simulink model "JointSpaceControl_own_MCP"  (R2013a)
settings: Solver=ode45  StartTime=0.0  StopTime=sim_end  MaxStep=0.008  RelTol=1e-3
PreLoadFcn:
  | Initialization
InitFcn:
  | Initialization
values from neighbouring files (symbols this model uses):
  a_max = [27 27 27 27 27 27]    [Initialization.m]
  dq_0 = qd_actual.signals.values(1,:)    [Initialization.m]
  K_0 = [            omega_1, zeros(1,5);         0,          omega_2, zeros(1,4);         zeros(1,2), omega_3, zeros(1,3);         zeros(1,3), omega_4, zeros(1,2);         zeros(1,4), omega_5, 0;         zeros(1,5), omega_6]    [Initialization.m]
  K_1 = [            omega_7, zeros(1,5);         0,          omega_8, zeros(1,4);         zeros(1,2), omega_9, zeros(1,3);         zeros(1,3), omega_10, zeros(1,2);         zeros(1,4), omega_11, 0;         zeros(1,5), omega_12]    [Initialization.m]
  q_0 = q_actual.signals.values(1,:)    [Initialization.m]
  q_max = 2*pi*ones(1,6)    [Initialization.m]
  q_min = -2*pi*ones(1,6)    [Initialization.m]
  torque_max = [150 150 150 28 28 28]    [Initialization.m]
  v_max = 3.4*ones(1,6)    [Initialization.m]
(part 2 of 4)

== matlab function JointSpaceControl_own_MCP/Forward & Velocity Kinematics Joint -> Tool Geometric Jacobian/J (made by Kathi) ==
  data: J output; q input; J1 output; J2 output
function [J, J1, J2]    = Jacobian(q)
% JACOBIAN - Jacobian from Base to Tool.
%  Calculates the Base-Tool Transformation matrix based on the current
%  joint positions and returns the rotation matrix and the displacement
%  vector.

theta_1 = q(1);
theta_2 = q(2);
theta_3 = q(3);
theta_4 = q(4);
theta_5 = q(5);
theta_6 = q(6);

J = [(109*cos(theta_1))/1000 + (41*cos(theta_1)*cos(theta_5))/500 + ...
        (17*cos(theta_2)*sin(theta_1))/40 - ...
        (93*cos(theta_4)*(cos(theta_2)*sin(theta_1)*sin(theta_3) + ...
        cos(theta_3)*sin(theta_1)*sin(theta_2)))/1000 + ...
        (93*sin(theta_4)*(sin(theta_1)*sin(theta_2)*sin(theta_3) - ...
        cos(theta_2)*cos(theta_3)*sin(theta_1)))/1000 - ...
        (41*sin(theta_5)*(cos(theta_4)*(sin(theta_1)*sin(theta_2)*sin(theta_3) - ...
        cos(theta_2)*cos(theta_3)*sin(theta_1)) + ...
        sin(theta_4)*(cos(theta_2)*sin(theta_1)*sin(theta_3) + ...
        cos(theta_3)*sin(theta_1)*sin(theta_2))))/500 - ...
        (39243*sin(theta_1)*sin(theta_2)*sin(theta_3))/100000 + ...
        (39243*cos(theta_2)*cos(theta_3)*sin(theta_1))/100000, ...
        ...
        (17*cos(theta_1)*sin(theta_2))/40 - ...
        (93*cos(theta_4)*(cos(theta_1)*sin(theta_2)*sin(theta_3) - ...
        cos(theta_1)*cos(theta_2)*cos(theta_3)))/1000 - ...
        (93*sin(theta_4)*(cos(theta_1)*cos(theta_2)*sin(theta_3) + ...
        cos(theta_1)*cos(theta_3)*sin(theta_2)))/1000 + ...
        (41*sin(theta_5)*(cos(theta_4)*(cos(theta_1)*cos(theta_2)*sin(theta_3) + ...
        cos(theta_1)*cos(theta_3)*sin(theta_2)) - ...
        sin(theta_4)*(cos(theta_1)*sin(theta_2)*sin(theta_3) - ...
        cos(theta_1)*cos(theta_2)*cos(theta_3))))/500 + ...
        (39243*cos(theta_1)*cos(theta_2)*sin(theta_3))/100000 + ...
        (39243*cos(theta_1)*cos(theta_3)*sin(theta_2))/100000, ...
        ...
        (41*sin(theta_5)*(cos(theta_4)*(cos(theta_1)*cos(theta_2)*sin(theta_3) + ...
        cos(theta_1)*cos(theta_3)*sin(theta_2)) - ...
        sin(theta_4)*(cos(theta_1)*sin(theta_2)*sin(theta_3) - ...
        cos(theta_1)*cos(theta_2)*cos(theta_3))))/500 - ...
        (93*sin(theta_4)*(cos(theta_1)*cos(theta_2)*sin(theta_3) + ...
        cos(theta_1)*cos(theta_3)*sin(theta_2)))/1000 - ...
        (93*cos(theta_4)*(cos(theta_1)*sin(theta_2)*sin(theta_3) - ...
        cos(theta_1)*cos(theta_2)*cos(theta_3)))/1000 + ...
        (39243*cos(theta_1)*cos(theta_2)*sin(theta_3))/100000 + ...
        (39243*cos(theta_1)*cos(theta_3)*sin(theta_2))/100000, ...
        ...
        (41*sin(theta_5)*(cos(theta_4)*(cos(theta_1)*cos(theta_2)*sin(theta_3) + ...
        cos(theta_1)*cos(theta_3)*sin(theta_2)) - ...
        sin(theta_4)*(cos(theta_1)*sin(theta_2)*sin(theta_3) - ...
        cos(theta_1)*cos(theta_2)*cos(theta_3))))/500 - ...
        (93*sin(theta_4)*(cos(theta_1)*cos(theta_2)*sin(theta_3) + ...
        cos(theta_1)*cos(theta_3)*sin(theta_2)))/1000 - ...
        (93*cos(theta_4)*(cos(theta_1)*sin(theta_2)*sin(theta_3) - ...
        cos(theta_1)*cos(theta_2)*cos(theta_3)))/1000, ...
        ...
        (41*cos(theta_5)*(cos(theta_4)*(cos(theta_1)*sin(theta_2)*sin(theta_3) - ...
        cos(theta_1)*cos(theta_2)*cos(theta_3)) + ...
        sin(theta_4)*(cos(theta_1)*cos(theta_2)*sin(theta_3) + ...
        cos(theta_1)*cos(theta_3)*sin(theta_2))))/500 - ...
        (41*sin(theta_1)*sin(theta_5))/500,... 
        ...
        0; ...
   (109*sin(theta_1))/1000 - (17*cos(theta_1)*cos(theta_2))/40 + ...
        (41*cos(theta_5)*sin(theta_1))/500 + ...
        (93*cos(theta_4)*(cos(theta_1)*cos(theta_2)*sin(theta_3) + ...
        cos(theta_1)*cos(theta_3)*sin(theta_2)))/1000 - ...
        (93*sin(theta_4)*(cos(theta_1)*sin(theta_2)*sin(theta_3) - ... 
        cos(theta_1)*cos(theta_2)*cos(theta_3)))/1000 + ...
        (41*sin(theta_5)*(cos(theta_4)*(cos(theta_1)*sin(theta_2)*sin(theta_3) - ...
        cos(theta_1)*cos(theta_2)*cos(theta_3)) + ...
        sin(theta_4)*(cos(theta_1)*cos(theta_2)*sin(theta_3) + ...
        cos(theta_1)*cos(theta_3)*sin(theta_2))))/500 + ...
        (39243*cos(theta_1)*sin(theta_2)*sin(theta_3))/100000 - ...
        (39243*cos(theta_1)*cos(theta_2)*cos(theta_3))/100000, ...
        ...
        (17*sin(theta_1)*sin(theta_2))/40 - ...
        (93*cos(theta_4)*(sin(theta_1)*sin(theta_2)*sin(theta_3) - ...
        cos(theta_2)*cos(theta_3)*sin(theta_1)))/1000 - ...
        (93*sin(theta_4)*(cos(theta_2)*sin(theta_1)*sin(theta_3) + ...
        cos(theta_3)*sin(theta_1)*sin(theta_2)))/1000 + ...
        (41*sin(theta_5)*(cos(theta_4)*(cos(theta_2)*sin(theta_1)*sin(theta_3) + ...
        cos(theta_3)*sin(theta_1)*sin(theta_2)) - ...
        sin(theta_4)*(sin(theta_1)*sin(theta_2)*sin(theta_3) - ...
        cos(theta_2)*cos(theta_3)*sin(theta_1))))/500 + ...
        (39243*cos(theta_2)*sin(theta_1)*sin(theta_3))/100000 + ...
        (39243*cos(theta_3)*sin(theta_1)*sin(theta_2))/100000, ...
        ...
        (41*sin(theta_5)*(cos(theta_4)*(cos(theta_2)*sin(theta_1)*sin(theta_3) + ...
        cos(theta_3)*sin(theta_1)*sin(theta_2)) - ...
        sin(theta_4)*(sin(theta_1)*sin(theta_2)*sin(theta_3) - ...
        cos(theta_2)*cos(theta_3)*sin(theta_1))))/500 - ...
        (93*sin(theta_4)*(cos(theta_2)*sin(theta_1)*sin(theta_3) + ...
        cos(theta_3)*sin(theta_1)*sin(theta_2)))/1000 - ...
        (93*cos(theta_4)*(sin(theta_1)*sin(theta_2)*sin(theta_3) - ...
        cos(theta_2)*cos(theta_3)*sin(theta_1)))/1000 + ...
        (39243*cos(theta_2)*sin(theta_1)*sin(theta_3))/100000 + ...
        (39243*cos(theta_3)*sin(theta_1)*sin(theta_2))/100000, ...
        ...
        (41*sin(theta_5)*(cos(theta_4)*(cos(theta_2)*sin(theta_1)*sin(theta_3) + ...
        cos(theta_3)*sin(theta_1)*sin(theta_2)) - ...
        sin(theta_4)*(sin(theta_1)*sin(theta_2)*sin(theta_3) - ...
        cos(theta_2)*cos(theta_3)*sin(theta_1))))/500 - ...
        (93*sin(theta_4)*(cos(theta_2)*sin(theta_1)*sin(theta_3) + ...
        cos(theta_3)*sin(theta_1)*sin(theta_2)))/1000 - ...
        (93*cos(theta_4)*(sin(theta_1)*sin(theta_2)*sin(theta_3) - ...
        cos(theta_2)*cos(theta_3)*sin(theta_1)))/1000, ...
        ...
        (41*cos(theta_1)*sin(theta_5))/500 + ...
        (41*cos(theta_5)*(cos(theta_4)*(sin(theta_1)*sin(theta_2)*sin(theta_3) - ...
        cos(theta_2)*cos(theta_3)*sin(theta_1)) + ...
        sin(theta_4)*(cos(theta_2)*sin(theta_1)*sin(theta_3) + ...
        cos(theta_3)*sin(theta_1)*sin(theta_2))))/500, ...
        ...
        0; ...
    0, ...
        ...
        (39243*sin(theta_2)*sin(theta_3))/100000 - ...
        (39243*cos(theta_2)*cos(theta_3))/100000 - ...
        (17*cos(theta_2))/40 - ...
        (41*sin(theta_5)*(cos(theta_4)*(cos(theta_2)*cos(theta_3) - ...
        sin(theta_2)*sin(theta_3)) - sin(theta_4)*(cos(theta_2)*sin(theta_3) + ...
        cos(theta_3)*sin(theta_2))))/500 + ...
        (93*cos(theta_4)*(cos(theta_2)*sin(theta_3) + ...
        cos(theta_3)*sin(theta_2)))/1000 + ...
        (93*sin(theta_4)*(cos(theta_2)*cos(theta_3) - sin(theta_2)*sin(theta_3)))/1000,...
        ...
        (39243*sin(theta_2)*sin(theta_3))/100000 - ...
        (39243*cos(theta_2)*cos(theta_3))/100000 - ...
        (41*sin(theta_5)*(cos(theta_4)*(cos(theta_2)*cos(theta_3) - ...
        sin(theta_2)*sin(theta_3)) - sin(theta_4)*(cos(theta_2)*sin(theta_3) + ...
        cos(theta_3)*sin(theta_2))))/500 + (93*cos(theta_4)*(cos(theta_2)*sin(theta_3) + ...
        cos(theta_3)*sin(theta_2)))/1000 + (93*sin(theta_4)*(cos(theta_2)*cos(theta_3) - ...
        sin(theta_2)*sin(theta_3)))/1000, ...
        ...
        (93*cos(theta_4)*(cos(theta_2)*sin(theta_3) + cos(theta_3)*sin(theta_2)))/1000 - ...
        (41*sin(theta_5)*(cos(theta_4)*(cos(theta_2)*cos(theta_3) - ...
        sin(theta_2)*sin(theta_3)) - sin(theta_4)*(cos(theta_2)*sin(theta_3) + ...
        cos(theta_3)*sin(theta_2))))/500 + (93*sin(theta_4)*(cos(theta_2)*cos(theta_3) - ...
        sin(theta_2)*sin(theta_3)))/1000,  ...
        ...
        -(41*cos(theta_5)*(cos(theta_4)*(cos(theta_2)*sin(theta_3) + ...
        cos(theta_3)*sin(theta_2)) + sin(theta_4)*(cos(theta_2)*cos(theta_3) - ...
        sin(theta_2)*sin(theta_3))))/500,  ...
        ...
        0; ...
    0, ...
        ...
        sin(theta_1), ...
        ...
        sin(theta_1), ...
        ...
        sin(theta_1), ...
        ...
        cos(theta_4)*(cos(theta_1)*cos(theta_2)*sin(theta_3) + ...
        cos(theta_1)*cos(theta_3)*sin(theta_2)) - ...
        sin(theta_4)*(cos(theta_1)*sin(theta_2)*sin(theta_3) - ...
        cos(theta_1)*cos(theta_2)*cos(theta_3)), ...
        ...
        cos(theta_5)*sin(theta_1) + ...
        sin(theta_5)*(cos(theta_4)*(cos(theta_1)*sin(theta_2)*sin(theta_3) - ...
        cos(theta_1)*cos(theta_2)*cos(theta_3)) + ...
        sin(theta_4)*(cos(theta_1)*cos(theta_2)*sin(theta_3) + ...
        cos(theta_1)*cos(theta_3)*sin(theta_2)));...
    0, ...
        ...
        -cos(theta_1), ...
        ...
        -cos(theta_1), ...
        ...
        -cos(theta_1), ...
        ...
        cos(theta_4)*(cos(theta_2)*sin(theta_1)*sin(theta_3) + ...
        cos(theta_3)*sin(theta_1)*sin(theta_2)) - ...
        sin(theta_4)*(sin(theta_1)*sin(theta_2)*sin(theta_3) - ...
        cos(theta_2)*cos(theta_3)*sin(theta_1)), ...
        ...
        sin(theta_5)*(cos(theta_4)*(sin(theta_1)*sin(theta_2)*sin(theta_3) - ...
        cos(theta_2)*cos(theta_3)*sin(theta_1)) + ...
        sin(theta_4)*(cos(theta_2)*sin(theta_1)*sin(theta_3) + ...
        cos(theta_3)*sin(theta_1)*sin(theta_2))) - cos(theta_1)*cos(theta_5);
    1, ...
        ...
        0, ...
        ...
        0, ...
        ...
        0, ...
        ...
        sin(theta_4)*(cos(theta_2)*sin(theta_3) + cos(theta_3)*sin(theta_2)) - ...
        cos(theta_4)*(cos(theta_2)*cos(theta_3) - sin(theta_2)*sin(theta_3)),...
        ...
        -sin(theta_5)*(cos(theta_4)*(cos(theta_2)*sin(theta_3) + ...
        cos(theta_3)*sin(theta_2)) + sin(theta_4)*(cos(theta_2)*cos(theta_3) - ...
        sin(theta_2)*sin(theta_3)));];
    J1 = J(1:6,1:3);
    J2 = J(1:6,4:6); 

end

== matlab function JointSpaceControl_own_MCP/Forward & Velocity Kinematics Joint -> Tool Geometric Jacobian/J_a ==
  data: J_a output; q input; theta input; phi input; psi input
function J_a     = Analytical_Jacobian(q, theta, phi, psi)
% ANALYTICAL JACOBIAN - Jacobian from Base to Tool.
%  Calculates the analytical Jacobian, based on the Euler angle transform
%  representation.

theta_1 = q(1);
theta_2 = q(2);
theta_3 = q(3);
theta_4 = q(4);
theta_5 = q(5);
theta_6 = q(6);

J = [(109*cos(theta_1))/1000 + (41*cos(theta_1)*cos(theta_5))/500 + ...
        (17*cos(theta_2)*sin(theta_1))/40 - ...
        (93*cos(theta_4)*(cos(theta_2)*sin(theta_1)*sin(theta_3) + ...
        cos(theta_3)*sin(theta_1)*sin(theta_2)))/1000 + ...
        (93*sin(theta_4)*(sin(theta_1)*sin(theta_2)*sin(theta_3) - ...
        cos(theta_2)*cos(theta_3)*sin(theta_1)))/1000 - ...
        (41*sin(theta_5)*(cos(theta_4)*(sin(theta_1)*sin(theta_2)*sin(theta_3) - ...
        cos(theta_2)*cos(theta_3)*sin(theta_1)) + ...
        sin(theta_4)*(cos(theta_2)*sin(theta_1)*sin(theta_3) + ...
        cos(theta_3)*sin(theta_1)*sin(theta_2))))/500 - ...
        (39243*sin(theta_1)*sin(theta_2)*sin(theta_3))/100000 + ...
        (39243*cos(theta_2)*cos(theta_3)*sin(theta_1))/100000, ...
        ...
        (17*cos(theta_1)*sin(theta_2))/40 - ...
        (93*cos(theta_4)*(cos(theta_1)*sin(theta_2)*sin(theta_3) - ...
        cos(theta_1)*cos(theta_2)*cos(theta_3)))/1000 - ...
        (93*sin(theta_4)*(cos(theta_1)*cos(theta_2)*sin(theta_3) + ...
        cos(theta_1)*cos(theta_3)*sin(theta_2)))/1000 + ...
        (41*sin(theta_5)*(cos(theta_4)*(cos(theta_1)*cos(theta_2)*sin(theta_3) + ...
        cos(theta_1)*cos(theta_3)*sin(theta_2)) - ...
        sin(theta_4)*(cos(theta_1)*sin(theta_2)*sin(theta_3) - ...
        cos(theta_1)*cos(theta_2)*cos(theta_3))))/500 + ...
        (39243*cos(theta_1)*cos(theta_2)*sin(theta_3))/100000 + ...
        (39243*cos(theta_1)*cos(theta_3)*sin(theta_2))/100000, ...
        ...
        (41*sin(theta_5)*(cos(theta_4)*(cos(theta_1)*cos(theta_2)*sin(theta_3) + ...
        cos(theta_1)*cos(theta_3)*sin(theta_2)) - ...
        sin(theta_4)*(cos(theta_1)*sin(theta_2)*sin(theta_3) - ...
        cos(theta_1)*cos(theta_2)*cos(theta_3))))/500 - ...
        (93*sin(theta_4)*(cos(theta_1)*cos(theta_2)*sin(theta_3) + ...
        cos(theta_1)*cos(theta_3)*sin(theta_2)))/1000 - ...
        (93*cos(theta_4)*(cos(theta_1)*sin(theta_2)*sin(theta_3) - ...
        cos(theta_1)*cos(theta_2)*cos(theta_3)))/1000 + ...
        (39243*cos(theta_1)*cos(theta_2)*sin(theta_3))/100000 + ...
        (39243*cos(theta_1)*cos(theta_3)*sin(theta_2))/100000, ...
        ...
        (41*sin(theta_5)*(cos(theta_4)*(cos(theta_1)*cos(theta_2)*sin(theta_3) + ...
        cos(theta_1)*cos(theta_3)*sin(theta_2)) - ...
        sin(theta_4)*(cos(theta_1)*sin(theta_2)*sin(theta_3) - ...
        cos(theta_1)*cos(theta_2)*cos(theta_3))))/500 - ...
        (93*sin(theta_4)*(cos(theta_1)*cos(theta_2)*sin(theta_3) + ...
        cos(theta_1)*cos(theta_3)*sin(theta_2)))/1000 - ...
        (93*cos(theta_4)*(cos(theta_1)*sin(theta_2)*sin(theta_3) - ...
        cos(theta_1)*cos(theta_2)*cos(theta_3)))/1000, ...
        ...
        (41*cos(theta_5)*(cos(theta_4)*(cos(theta_1)*sin(theta_2)*sin(theta_3) - ...
        cos(theta_1)*cos(theta_2)*cos(theta_3)) + ...
        sin(theta_4)*(cos(theta_1)*cos(theta_2)*sin(theta_3) + ...
        cos(theta_1)*cos(theta_3)*sin(theta_2))))/500 - ...
        (41*sin(theta_1)*sin(theta_5))/500,... 
        ...
        0; ...
   (109*sin(theta_1))/1000 - (17*cos(theta_1)*cos(theta_2))/40 + ...
        (41*cos(theta_5)*sin(theta_1))/500 + ...
        (93*cos(theta_4)*(cos(theta_1)*cos(theta_2)*sin(theta_3) + ...
        cos(theta_1)*cos(theta_3)*sin(theta_2)))/1000 - ...
        (93*sin(theta_4)*(cos(theta_1)*sin(theta_2)*sin(theta_3) - ... 
        cos(theta_1)*cos(theta_2)*cos(theta_3)))/1000 + ...
        (41*sin(theta_5)*(cos(theta_4)*(cos(theta_1)*sin(theta_2)*sin(theta_3) - ...
        cos(theta_1)*cos(theta_2)*cos(theta_3)) + ...
        sin(theta_4)*(cos(theta_1)*cos(theta_2)*sin(theta_3) + ...
        cos(theta_1)*cos(theta_3)*sin(theta_2))))/500 + ...
        (39243*cos(theta_1)*sin(theta_2)*sin(theta_3))/100000 - ...
        (39243*cos(theta_1)*cos(theta_2)*cos(theta_3))/100000, ...
        ...
        (17*sin(theta_1)*sin(theta_2))/40 - ...
        (93*cos(theta_4)*(sin(theta_1)*sin(theta_2)*sin(theta_3) - ...
        cos(theta_2)*cos(theta_3)*sin(theta_1)))/1000 - ...
        (93*sin(theta_4)*(cos(theta_2)*sin(theta_1)*sin(theta_3) + ...
        cos(theta_3)*sin(theta_1)*sin(theta_2)))/1000 + ...
        (41*sin(theta_5)*(cos(theta_4)*(cos(theta_2)*sin(theta_1)*sin(theta_3) + ...
        cos(theta_3)*sin(theta_1)*sin(theta_2)) - ...
        sin(theta_4)*(sin(theta_1)*sin(theta_2)*sin(theta_3) - ...
        cos(theta_2)*cos(theta_3)*sin(theta_1))))/500 + ...
        (39243*cos(theta_2)*sin(theta_1)*sin(theta_3))/100000 + ...
        (39243*cos(theta_3)*sin(theta_1)*sin(theta_2))/100000, ...
        ...
        (41*sin(theta_5)*(cos(theta_4)*(cos(theta_2)*sin(theta_1)*sin(theta_3) + ...
        cos(theta_3)*sin(theta_1)*sin(theta_2)) - ...
        sin(theta_4)*(sin(theta_1)*sin(theta_2)*sin(theta_3) - ...
        cos(theta_2)*cos(theta_3)*sin(theta_1))))/500 - ...
        (93*sin(theta_4)*(cos(theta_2)*sin(theta_1)*sin(theta_3) + ...
        cos(theta_3)*sin(theta_1)*sin(theta_2)))/1000 - ...
        (93*cos(theta_4)*(sin(theta_1)*sin(theta_2)*sin(theta_3) - ...
        cos(theta_2)*cos(theta_3)*sin(theta_1)))/1000 + ...
        (39243*cos(theta_2)*sin(theta_1)*sin(theta_3))/100000 + ...
        (39243*cos(theta_3)*sin(theta_1)*sin(theta_2))/100000, ...
        ...
        (41*sin(theta_5)*(cos(theta_4)*(cos(theta_2)*sin(theta_1)*sin(theta_3) + ...
        cos(theta_3)*sin(theta_1)*sin(theta_2)) - ...
        sin(theta_4)*(sin(theta_1)*sin(theta_2)*sin(theta_3) - ...
        cos(theta_2)*cos(theta_3)*sin(theta_1))))/500 - ...
        (93*sin(theta_4)*(cos(theta_2)*sin(theta_1)*sin(theta_3) + ...
        cos(theta_3)*sin(theta_1)*sin(theta_2)))/1000 - ...
        (93*cos(theta_4)*(sin(theta_1)*sin(theta_2)*sin(theta_3) - ...
        cos(theta_2)*cos(theta_3)*sin(theta_1)))/1000, ...
        ...
        (41*cos(theta_1)*sin(theta_5))/500 + ...
        (41*cos(theta_5)*(cos(theta_4)*(sin(theta_1)*sin(theta_2)*sin(theta_3) - ...
        cos(theta_2)*cos(theta_3)*sin(theta_1)) + ...
        sin(theta_4)*(cos(theta_2)*sin(theta_1)*sin(theta_3) + ...
        cos(theta_3)*sin(theta_1)*sin(theta_2))))/500, ...
        ...
        0; ...
    0, ...
        ...
        (39243*sin(theta_2)*sin(theta_3))/100000 - ...
        (39243*cos(theta_2)*cos(theta_3))/100000 - ...
        (17*cos(theta_2))/40 - ...
        (41*sin(theta_5)*(cos(theta_4)*(cos(theta_2)*cos(theta_3) - ...
        sin(theta_2)*sin(theta_3)) - sin(theta_4)*(cos(theta_2)*sin(theta_3) + ...
        cos(theta_3)*sin(theta_2))))/500 + ...
        (93*cos(theta_4)*(cos(theta_2)*sin(theta_3) + ...
        cos(theta_3)*sin(theta_2)))/1000 + ...
        (93*sin(theta_4)*(cos(theta_2)*cos(theta_3) - sin(theta_2)*sin(theta_3)))/1000,...
        ...
        (39243*sin(theta_2)*sin(theta_3))/100000 - ...
        (39243*cos(theta_2)*cos(theta_3))/100000 - ...
        (41*sin(theta_5)*(cos(theta_4)*(cos(theta_2)*cos(theta_3) - ...
        sin(theta_2)*sin(theta_3)) - sin(theta_4)*(cos(theta_2)*sin(theta_3) + ...
        cos(theta_3)*sin(theta_2))))/500 + (93*cos(theta_4)*(cos(theta_2)*sin(theta_3) + ...
        cos(theta_3)*sin(theta_2)))/1000 + (93*sin(theta_4)*(cos(theta_2)*cos(theta_3) - ...
        sin(theta_2)*sin(theta_3)))/1000, ...
        ...
        (93*cos(theta_4)*(cos(theta_2)*sin(theta_3) + cos(theta_3)*sin(theta_2)))/1000 - ...
        (41*sin(theta_5)*(cos(theta_4)*(cos(theta_2)*cos(theta_3) - ...
        sin(theta_2)*sin(theta_3)) - sin(theta_4)*(cos(theta_2)*sin(theta_3) + ...
        cos(theta_3)*sin(theta_2))))/500 + (93*sin(theta_4)*(cos(theta_2)*cos(theta_3) - ...
        sin(theta_2)*sin(theta_3)))/1000,  ...
        ...
        -(41*cos(theta_5)*(cos(theta_4)*(cos(theta_2)*sin(theta_3) + ...
        cos(theta_3)*sin(theta_2)) + sin(theta_4)*(cos(theta_2)*cos(theta_3) - ...
        sin(theta_2)*sin(theta_3))))/500,  ...
        ...
        0; ...
    0, ...
        ...
        sin(theta_1), ...
        ...
        sin(theta_1), ...
        ...
        sin(theta_1), ...
        ...
        cos(theta_4)*(cos(theta_1)*cos(theta_2)*sin(theta_3) + ...
        cos(theta_1)*cos(theta_3)*sin(theta_2)) - ...
        sin(theta_4)*(cos(theta_1)*sin(theta_2)*sin(theta_3) - ...
        cos(theta_1)*cos(theta_2)*cos(theta_3)), ...
        ...
        cos(theta_5)*sin(theta_1) + ...
        sin(theta_5)*(cos(theta_4)*(cos(theta_1)*sin(theta_2)*sin(theta_3) - ...
        cos(theta_1)*cos(theta_2)*cos(theta_3)) + ...
        sin(theta_4)*(cos(theta_1)*cos(theta_2)*sin(theta_3) + ...
        cos(theta_1)*cos(theta_3)*sin(theta_2)));...
    0, ...
        ...
        -cos(theta_1), ...
        ...
        -cos(theta_1), ...
        ...
        -cos(theta_1), ...
        ...
        cos(theta_4)*(cos(theta_2)*sin(theta_1)*sin(theta_3) + ...
        cos(theta_3)*sin(theta_1)*sin(theta_2)) - ...
        sin(theta_4)*(sin(theta_1)*sin(theta_2)*sin(theta_3) - ...
        cos(theta_2)*cos(theta_3)*sin(theta_1)), ...
        ...
        sin(theta_5)*(cos(theta_4)*(sin(theta_1)*sin(theta_2)*sin(theta_3) - ...
        cos(theta_2)*cos(theta_3)*sin(theta_1)) + ...
        sin(theta_4)*(cos(theta_2)*sin(theta_1)*sin(theta_3) + ...
        cos(theta_3)*sin(theta_1)*sin(theta_2))) - cos(theta_1)*cos(theta_5);
    1, ...
        ...
        0, ...
        ...
        0, ...
        ...
        0, ...
        ...
        sin(theta_4)*(cos(theta_2)*sin(theta_3) + cos(theta_3)*sin(theta_2)) - ...
        cos(theta_4)*(cos(theta_2)*cos(theta_3) - sin(theta_2)*sin(theta_3)),...
        ...
        -sin(theta_5)*(cos(theta_4)*(cos(theta_2)*sin(theta_3) + ...
        cos(theta_3)*sin(theta_2)) + sin(theta_4)*(cos(theta_2)*cos(theta_3) - ...
        sin(theta_2)*sin(theta_3)));];

    B_alpha = [cos(psi)*sin(theta), -sin(psi), 0; ...
               sin(psi)*sin(theta), cos(psi), 0; ...
               cos(theta), 0, 1];
    Transf = [eye(3,3), zeros(3,3); zeros(3,3), inv(B_alpha)];
    J_a = Transf*J;

end

== matlab function JointSpaceControl_own_MCP/Convert to axis//angle representation (same form as used by the model)1/R_to_axis_angle ==
  data: R input; k output; theta output
function [k, theta]  = R_to_axis_angle(R)
% R_TO_AXIS_ANGLE Transform the transformation matrix representation to the
% axis/angle representation.
 theta = (cos((R(1,1)+R(2,2)+R(3,3)-1)/2))^(-1);
 k = 1/(2*sin(theta))*[R(3,2)-R(2,3); R(1,3)-R(3,1); R(2,1)-R(1,2)];
end

== matlab function JointSpaceControl_own_MCP/Convert to axis//angle representation (same form as used by the model)1/R_to_axis_angle1 ==
  data: R input; k output; theta output
function [k, theta]  = R_to_axis_angle(R)
% R_TO_AXIS_ANGLE Transform the transformation matrix representation to the
% axis/angle representation.
 theta = acos((R(1,1)+R(2,2)+R(3,3)-1)/2);
 k = 1/(2*sin(theta))*[R(3,2)-R(2,3); R(1,3)-R(3,1); R(2,1)-R(1,2)];
end

== matlab function JointSpaceControl_own_MCP/Convert to axis//angle representation (same form as used by the model)1/RxRyRz to axis angle ==
  data: RxRyRz input; k output; theta output
function [k, theta]  = RxRyRz_to_k_theta(RxRyRz)
% RXRYRZ_TO_K_THETA Transform the RxRyRz representation to the axis/angle
% representation
 theta = norm(RxRyRz);
 k = RxRyRz/theta;
end

== matlab function JointSpaceControl_own_MCP/Convert to axis//angle representation (same form as used by the model)1/axis angle to transformation matrix ==
  data: k input; theta input; R output
function R   = axis_angle_to_R(k, theta)
% AXIS_ANGLE_TO_R Transform the axis/angle representation to a rotation
% matrix representation.
kx = k(1);
ky = k(2);
kz = k(3);

v = 1-cos(theta);
s = sin(theta);
c = cos (theta);

r11 = kx^2*v + c;
r12 = kx*ky*v - kz*s;
r13 = kx*kz*v+ky*s;
r21 = kx*ky*v+kz*s;
r22 = ky^2*v + c;
r23 = ky*kz*v-kx*s;
r31 = kx*kz*v-ky*s;
r32 = ky*kz*v + kx*s;
r33 = kz^2*v+c;

R = [r11, r12, r13; r21, r22, r23; r31, r32, r33];

end
